simulink model "exSyncGenPVinv_sim"  (R2014b)
settings: Solver=ode45  SolverMode=SingleTasking  StartTime=0.0  StopTime=20  MaxStep=0.002  RelTol=1e-07
values from neighbouring files (symbols this model uses):
  bus1_vd = 2^0.5*1e3    (= 1414.21356237)    [ex3busPV.m]    (also in exLongLinePV.m = 141421.356237)
  Cbus_ext = 1e6*mpcC.bus(ssgen,BS)./(ws*baseV(ssgen).^2)    [exDroopA.m]    (also in exDroopB.m; exSyncGenPVinv.m)
  Cbuseff = 2*Ebus/Vdcset^2    [exSyncGenPVinv.m]
  droop_D = 5e-4*(2/poles)./J    [exSyncGenPVinv.m]
  droop_Pref = 0.25*Pbase    (= 75000000)    [ex7busLongLine.m]    (also in exDroopA.m = mpc.gen(2:end,PG)*1e6; exDroopB.m = mpc.gen(:,PG)*1e6; exSyncGenPVinv.m = droop_Pref( [1:(synrp-1),(synrp+1):end]  ))
  If_dc = 0.2*Prt./Ert    [ex14busSGandPV.m]    (also in ex7busLongLine.m = Prt./(60*Vf_dc); exDroopA.m = Prt./(60*Vf_dc); exDroopB.m = Prt./(60*Vf_dc); exSyncGenPVinv.m)
  Kci = Kcp^2/(2*Linv)    [exSyncGenPVinv.m]    (also in pv_dq.m = 3.11562907794)
  Kcp = 10*4*pi*Linv    [exSyncGenPVinv.m]    (also in pv_dq.m = 0.0495867768595)
  Kpi = 0.1*Kpp^2/(Ebus/Vinv_rt)    [exSyncGenPVinv.m]    (also in pv_dq.m = 251.934662919)
  Kpp = 200*(Ebus/Vinv_rt)    [exSyncGenPVinv.m]    (also in pv_dq.m = 12.596733146)
  L0 = 0.1*Ld    [ex14busSGandPV.m]    (also in ex7busLongLine.m; exDroopA.m; exDroopB.m; exSyncGenPVinv.m)
  Laf = (2^0.5)*Ert./(ws*If_dc)    [ex14busSGandPV.m]    (also in ex7busLongLine.m; exDroopA.m; exDroopB.m; exSyncGenPVinv.m = (2^0.5)*5*Ert.^2./(ws*Prt))
  Lb2 = 2*Ld.*Lff - 3*Laf.^2    [ex14busSGandPV.m]    (also in ex7busLongLine.m; exDroopA.m; exDroopB.m; exSyncGenPVinv.m)
  Ld = 0.6*Lpu    [ex14busSGandPV.m]    (also in ex7busLongLine.m = 0.3*Lpu; exDroopA.m = 0.3*Lpu; exDroopB.m = 0.3*Lpu; exSyncGenPVinv.m)
  Lff = 2*Laf.^2./Ld    [ex14busSGandPV.m]    (also in ex7busLongLine.m; exDroopA.m; exDroopB.m; exSyncGenPVinv.m)
  Linv = 10*(1/ws)*Pinv_rt/Vinv_rt^2    [exSyncGenPVinv.m]
  Lq = Ld    [ex14busSGandPV.m]    (also in ex7busLongLine.m; exDroopA.m; exDroopB.m; exSyncGenPVinv.m)
  nG = length(ssgen)    [exDroopA.m]    (also in exSyncGenPVinv.m)
  Pdc_op = 0.6*Pinv_rt    [exSyncGenPVinv.m]    (also in pv_dq.m = 1600000)
  poles_2Jws = poles./(2*J*ws)    [ex14busSGandPV.m]    (also in ex2busStability.m = poles./(2*ws*J); ex7busLongLine.m; ex9busSG.m = poles./(2*ws*J); exDroopA.m)
  Qstar = 0    [exSyncGenPVinv.m]    (also in pv_dq.m)
  Ra = 0.05*Ert.^2./Prt    [ex14busSGandPV.m]    (also in ex7busLongLine.m = 0.01*Ert.^2./Prt; exDroopA.m = 0.01*Ert.^2./Prt; exDroopB.m = 0.01*Ert.^2./Prt; exSyncGenPVinv.m)
  Rf = Lff/1.2    [ex14busSGandPV.m]    (also in ex7busLongLine.m = Vf_dc./If_dc; exDroopA.m = Vf_dc./If_dc; exDroopB.m = Vf_dc./If_dc; exSyncGenPVinv.m)
  synrp = 2    [exSyncGenPVinv.m]
  units_to_net = zeros(1,3*Nss)    [ex14busSGandPV.m]    (also in exDroopA.m = [1,4:(3+nG),2,(4+nG):(3+2*nG),3,(4+2*nG):(3+3*nG)]; exSyncGenPVinv.m = [1,4:(3+nG),2,(4+nG):(3+2*nG),3,(4+2*nG):(3+3*nG)])
  vcap_init_0 = 0*vppa    [exDroopA.m]    (also in exDroopB.m; exSyncGenPVinv.m)
  vcap_init_d = real(vppa)    [exDroopA.m]    (also in exDroopB.m; exSyncGenPVinv.m)
  vcap_init_q = imag(vppa)    [exDroopA.m]    (also in exDroopB.m; exSyncGenPVinv.m)
  Vdcset = (2^0.5)*Vinv_rt/duty_max    [exSyncGenPVinv.m]    (also in pv_dq.m = 19958.8053116)
  Vf_dc = If_dc.*Rf    [ex14busSGandPV.m]    (also in ex7busLongLine.m = 500 * ones(size(Ert)); exDroopA.m = 500 * ones(size(Ert)); exDroopB.m = 500 * ones(size(Ert)); exSyncGenPVinv.m)
  vinf_0 = 0    [ex14busSGandPV.m]    (also in ex7busLongLine.m; exDroopA.m; exSyncGenPVinv.m)
  vinf_d = (2^0.5)*mpcA.bus(1,VM)*baseV    [ex14busSGandPV.m]    (also in ex7busLongLine.m = 250457.221896; exDroopA.m = (2^0.5)*mpc.bus(1,VM)*baseV(1); exSyncGenPVinv.m = (2^0.5)*mpc.bus(1,VM)*baseV(1))
  vinf_q = 0    [ex14busSGandPV.m]    (also in ex7busLongLine.m; exDroopA.m; exSyncGenPVinv.m)
  Vinv_rt = mpc.bus(ssgen(synrp),VM).*baseV(ssgen(synrp))    [exSyncGenPVinv.m]    (also in pv_dq.m = 12701.7059222)
  ws = 2*pi*50    (= 314.159265359)    [ex14busSGandPV.m]    (also in ex2busStability.m; ex3busPV.m; ex7busLongLine.m; ex9busSG.m)
undefined symbols (not defined in the file or in its folder): Anet, Bnet, Cnet, Dnet, full, magnitude, net_to_units
libraries: simulink x1
settings Model: Creator=COPEC  LastModifiedBy=yoashl
settings OptimizationCC: BlockReduction=off  BooleanDataType=off
settings DebuggingCC: SaveWithParameterizedLinksMsg=none  UnderspecifiedInitializationDetection=Classic  MergeDetectMultiDrivingBlocksExec=none  SignalResolutionControl=TryResolveAllWithWarning  SolverPrmCheckMsg=none  FrameProcessingCompatibilityMsg=error
settings HardwareCC: TargetUnknown=on

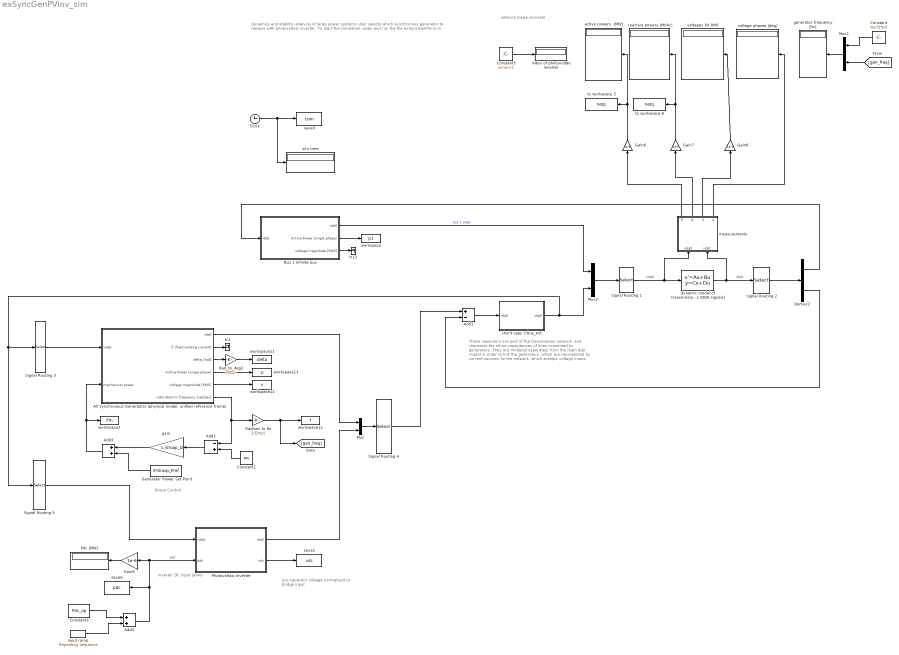
== system exSyncGenPVinv_sim ==
  note: Droop Control
  note: Dynamics and stability analysis of large power systems
      | User selects which synchronous generator to replace with photovoltaic inverter.
      |
      | To start the simulation, open and run the file
      | exSyncGenPVinv.m
  note: These capacitors are part of the transmission network, and represent the shunt capacitances of lines connected to generators. They are modeled seperately from the main dq0 model in order to link the generators, which are represented by current sources, to the network, which accepts voltage inputs.
  note: network measurements
  note: bus capacitor voltage normalized to bridge input
  note: inverter DC input power
  Add1 : Sum  Inputs=+-
  Add2 : Sum  Inputs=-+
  Add3 : Sum
  Add4 : Sum
  "All Synchronous Generators (physical model, unified reference frame)" : Subsystem
  Bus 1 Infinite bus : Subsystem
  Clock : Clock
  Constant : Constant  Value=ws/(2*pi)
  Constant1 : Constant  Value=ws
  Constant2 : Constant  Value=Pdc_op
  Constant3 : Constant  Value=synrp+1
  Demux2 : Demux  Outputs=[3 , length(net_to_units)-3]
  Gain6 : Gain  Gain=1e-6
  Gain7 : Gain  Gain=1e-6
  Gain8 : Gain  Gain=1e-3
  Gain9 : Gain  Gain=1e-6
  Generator Power Set Point : Constant  Value=3*droop_Pref
  Mux : Mux  Inputs=2
  Mux1 : Mux  Inputs=2
  Mux2 : Mux  Inputs=2
  Pdc [MW] : Display
  Photovoltaic Inverter : Subsystem
  Rad/sec to Hz : Gain  Gain=1/(2*pi)
  Rad_to_deg2 : Gain  Gain=180/pi
  Signal Routing 1 : Selector  InputPortWidth=length(units_to_net)  IndexOptions=Index vector (dialog)  Indices=units_to_net  OutputSizes=1
  Signal Routing 2 : Selector  InputPortWidth=length(net_to_units)  IndexOptions=Index vector (dialog)  Indices=net_to_units  OutputSizes=1
  Signal Routing 3 : Selector  InputPortWidth=3*nG  IndexOptions=Index vector (dialog)  Indices=routing1  OutputSizes=1
  Signal Routing 4 : Selector  InputPortWidth=3*nG  IndexOptions=Index vector (dialog)  Indices=routing3  OutputSizes=1
  Signal Routing 5 : Selector  InputPortWidth=3*nG  IndexOptions=Index vector (dialog)  Indices=routing2  OutputSizes=1
  active powers  [MW] : Display
  dynamic model of transmission network with integrated loads (DQ0 signals) : StateSpace  A=full(Anet)  B=full(Bnet)  C=full(Cnet)  D=full(Dnet)  X0=0
  gain : Gain  Gain=1./droop_D
  generator frequency [Hz] : Display
  index of photovoltaic inverter : Display
  input ramp : simulink/Sources/Repeating Sequence  rep_seq_t=[0 1 1e6]  rep_seq_y=[0 0 0]
  measurements : Subsystem
  reactive powers [MVAr] : Display
  save0 : ToWorkspace  VariableName=tsim  SampleTime=-1
  save2 : ToWorkspace  VariableName=vdc  SampleTime=-1
  save6 : ToWorkspace  VariableName=pdc  SampleTime=-1
  "shunt caps 'Cbus_ext' " : Subsystem
  sim time : Display
  to workspace 5 : ToWorkspace  VariableName=netp  SampleTime=-1
  to workspace 6 : ToWorkspace  VariableName=netq  SampleTime=-1
  tr12 : Terminator
  tr2 : Terminator
  voltage phases [deg] : Display
  voltages kV RMS : Display
  workspace : ToWorkspace  VariableName=p1  SampleTime=-1
  workspace1 : ToWorkspace  VariableName=Pm  SampleTime=-1
  workspace11 : ToWorkspace  VariableName=delta  SampleTime=-1
  workspace12 : ToWorkspace  VariableName=f  SampleTime=-1
  workspace13 : ToWorkspace  VariableName=p  SampleTime=-1
  workspace14 : ToWorkspace  VariableName=v  SampleTime=-1
  wires:
  Clock/1 -> sim time/1, save0/1
  Bus 1 Infinite bus/3(voltage magnitude [RMS]) -> tr12/1
  Bus 1 Infinite bus/2(Active Power (single phase)) -> workspace/1
  "All Synchronous Generators (physical model, unified reference frame)"/2(if (field winding current)) -> tr2/1
  "All Synchronous Generators (physical model, unified reference frame)"/3(delta_[rad]) -> Rad_to_deg2/1
  Rad_to_deg2/1 -> workspace11/1
  "All Synchronous Generators (physical model, unified reference frame)"/6(rotor electric frequency [rad/sec]) -> Rad/sec to Hz/1, Add2/1
  Rad/sec to Hz/1 -> workspace12/1, [gen_freq]
  "All Synchronous Generators (physical model, unified reference frame)"/4(Active Power (single phase)) -> workspace13/1
  "All Synchronous Generators (physical model, unified reference frame)"/5(voltage magnitude [RMS]) -> workspace14/1
  Add1/1 -> "shunt caps 'Cbus_ext' "/1(idq0)
  "shunt caps 'Cbus_ext' "/1(vdq0) -> Signal Routing 5/1, Signal Routing 3/1, Mux2/2
  Bus 1 Infinite bus/1(vdq0) -> Mux2/1  "bus 1 vdq0"
  Mux2/1 -> Signal Routing 1/1
  Signal Routing 1/1 -> measurements/1(vdq0), dynamic model of transmission network with integrated loads (DQ0 signals)/1  "vdq0"
  dynamic model of transmission network with integrated loads (DQ0 signals)/1 -> measurements/2(idq0), Signal Routing 2/1  "idq0"
  Signal Routing 2/1 -> Demux2/1
  Demux2/2 -> Add1/2
  Demux2/1 -> Bus 1 Infinite bus/1(idq0)
  Constant1/1 -> Add2/2
  Add2/1 -> gain/1
  Generator Power Set Point/1 -> Add3/2
  gain/1 -> Add3/1
  Add3/1 -> workspace1/1, "All Synchronous Generators (physical model, unified reference frame)"/2(mechanical power)
  Gain8/1 -> voltages kV RMS/1
  measurements/2(Q) -> Gain7/1
  Constant/1 -> Mux1/1
  Gain7/1 -> reactive powers [MVAr]/1, to workspace 6/1
  Mux1/1 -> generator frequency [Hz]/1
  measurements/3(Vm_RMS) -> Gain8/1
  measurements/4(Vph_deg) -> voltage phases [deg]/1
  Gain6/1 -> to workspace 5/1, active powers  [MW]/1
  [gen_freq] -> Mux1/2
  measurements/1(P) -> Gain6/1
  Photovoltaic Inverter/2(vdc) -> save2/1
  input ramp/1 -> Add4/2
  Add4/1 -> Photovoltaic Inverter/2(pdc), Gain9/1, save6/1  "pdc"
  Gain9/1 -> Pdc [MW]/1
  Constant2/1 -> Add4/1
  "All Synchronous Generators (physical model, unified reference frame)"/1(idq0) -> Mux/1
  Signal Routing 3/1 -> "All Synchronous Generators (physical model, unified reference frame)"/1(vdq0)
  Photovoltaic Inverter/1(idq0) -> Mux/2
  Mux/1 -> Signal Routing 4/1
  Signal Routing 4/1 -> Add1/1
  Signal Routing 5/1 -> Photovoltaic Inverter/1(vdq0)
  Constant3/1 -> index of photovoltaic inverter/1

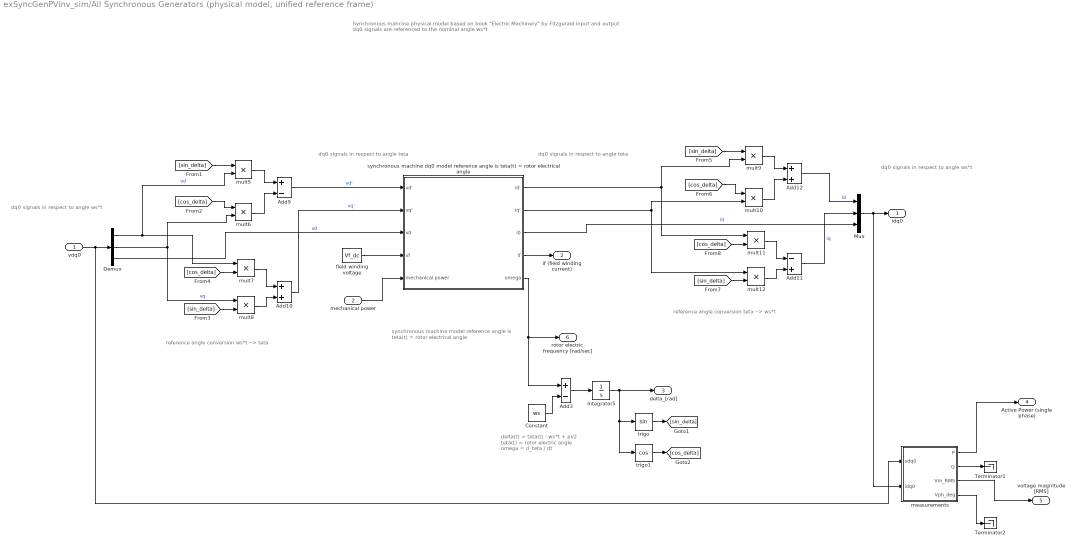
== system exSyncGenPVinv_sim/All Synchronous Generators (physical model, unified reference frame) ==
  note: Synchronous mahcine physical model
      | based on book "Electric Machinery" by Fitzgerald
      |
      | input and output dq0 signals are referenced
      | to the nominal angle ws*t
  note: reference angle conversion ws*t --> teta
  note: synchronous machine model
      | reference angle is
      | teta(t) = rotor electrical angle
  note: reference angle conversion teta --> ws*t
  note: dq0 signals in respect to angle ws*t
  note: dq0 signals in respect to angle ws*t
  note: dq0 signals in respect to angle teta
  note: dq0 signals in respect to angle teta
  note: delta(t) = teta(t) - ws*t + pi/2
      | teta(t) = rotor electric angle
      | omega = d_teta / dt
  vdq0 : Inport
  mechanical power : Inport  Port=2
  Add10 : Sum
  Add11 : Sum  Inputs=-+
  Add12 : Sum
  Add3 : Sum  Inputs=+-
  Add9 : Sum  Inputs=+-
  Constant : Constant  Value=ws
  Demux : Demux  Outputs=3
  Integrator5 : Integrator
  Mux : Mux  Inputs=3
  Terminator1 : Terminator
  Terminator2 : Terminator
  field winding voltage : Constant  Value=Vf_dc
  measurements : Subsystem
  mult{5..12} (8 alike) : Product  Inputs=**
  synchronous machine dq0 model reference angle is teta(t) = rotor electrical angle : Subsystem
  trigo : Trigonometry
  trigo1 : Trigonometry  Operator=cos
  idq0 : Outport
  if (field winding current) : Outport  Port=2
  delta_[rad] : Outport  Port=3
  Active Power (single phase) : Outport  Port=4
  voltage magnitude [RMS] : Outport  Port=5
  rotor electric frequency [rad/sec] : Outport  Port=6
  wires:
  vdq0/1 -> measurements/1(vdq0), Demux/1
  Demux/1 -> mult5/2, mult7/1  "vd"
  Demux/2 -> mult6/2, mult8/1  "vq"
  mult5/1 -> Add9/1
  mult6/1 -> Add9/2
  [sin_delta] -> mult5/1
  [cos_delta] -> mult6/1
  mult7/1 -> Add10/1
  mult8/1 -> Add10/2
  [cos_delta] -> mult7/2
  [sin_delta] -> mult8/2
  mult9/1 -> Add12/1
  mult10/1 -> Add12/2
  [sin_delta] -> mult9/1
  [cos_delta] -> mult10/1
  mult11/1 -> Add11/1
  mult12/1 -> Add11/2
  [cos_delta] -> mult11/2
  [sin_delta] -> mult12/2
  Mux/1 -> measurements/2(idq0), idq0/1
  Add11/1 -> Mux/2  "iq"
  Add12/1 -> Mux/1  "id"
  synchronous machine dq0 model reference angle is teta(t) = rotor electrical angle/1(id') -> mult11/1, mult9/2
  synchronous machine dq0 model reference angle is teta(t) = rotor electrical angle/2(iq') -> mult12/1, mult10/2
  Add9/1 -> synchronous machine dq0 model reference angle is teta(t) = rotor electrical angle/1(vd')  "vd'"
  mechanical power/1 -> synchronous machine dq0 model reference angle is teta(t) = rotor electrical angle/5(mechanical power)
  Demux/3 -> synchronous machine dq0 model reference angle is teta(t) = rotor electrical angle/3(v0)  "v0"
  Add10/1 -> synchronous machine dq0 model reference angle is teta(t) = rotor electrical angle/2(vq')  "vq'"
  field winding voltage/1 -> synchronous machine dq0 model reference angle is teta(t) = rotor electrical angle/4(vf)
  synchronous machine dq0 model reference angle is teta(t) = rotor electrical angle/3(i0) -> Mux/3  "i0"
  synchronous machine dq0 model reference angle is teta(t) = rotor electrical angle/4(if) -> if (field winding current)/1
  trigo/1 -> [sin_delta]
  trigo1/1 -> [cos_delta]
  Add3/1 -> Integrator5/1
  Constant/1 -> Add3/2
  synchronous machine dq0 model reference angle is teta(t) = rotor electrical angle/5(omega) -> Add3/1, rotor electric frequency [rad/sec]/1
  Integrator5/1 -> delta_[rad]/1, trigo1/1, trigo/1
  measurements/1(P) -> Active Power (single phase)/1
  measurements/2(Q) -> Terminator1/1
  measurements/3(Vm_RMS) -> voltage magnitude [RMS]/1
  measurements/4(Vph_deg) -> Terminator2/1

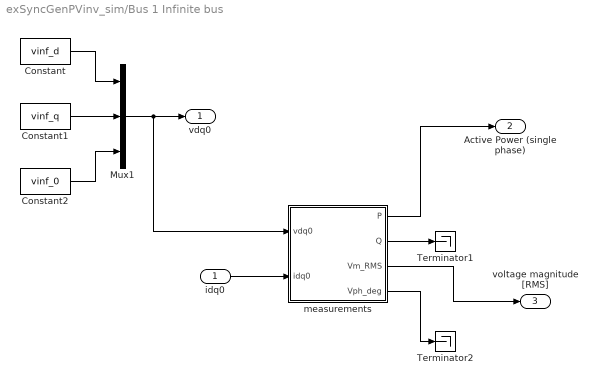
== system exSyncGenPVinv_sim/Bus 1 Infinite bus ==
  idq0 : Inport
  Constant : Constant  Value=vinf_d
  Constant1 : Constant  Value=vinf_q
  Constant2 : Constant  Value=vinf_0
  Mux1 : Mux  Inputs=3
  Terminator1 : Terminator
  Terminator2 : Terminator
  measurements : Subsystem
  vdq0 : Outport
  Active Power (single phase) : Outport  Port=2
  voltage magnitude [RMS] : Outport  Port=3
  wires:
  measurements/1(P) -> Active Power (single phase)/1
  measurements/2(Q) -> Terminator1/1
  measurements/3(Vm_RMS) -> voltage magnitude [RMS]/1
  measurements/4(Vph_deg) -> Terminator2/1
  idq0/1 -> measurements/2(idq0)
  Mux1/1 -> measurements/1(vdq0), vdq0/1
  Constant/1 -> Mux1/1
  Constant1/1 -> Mux1/2
  Constant2/1 -> Mux1/3

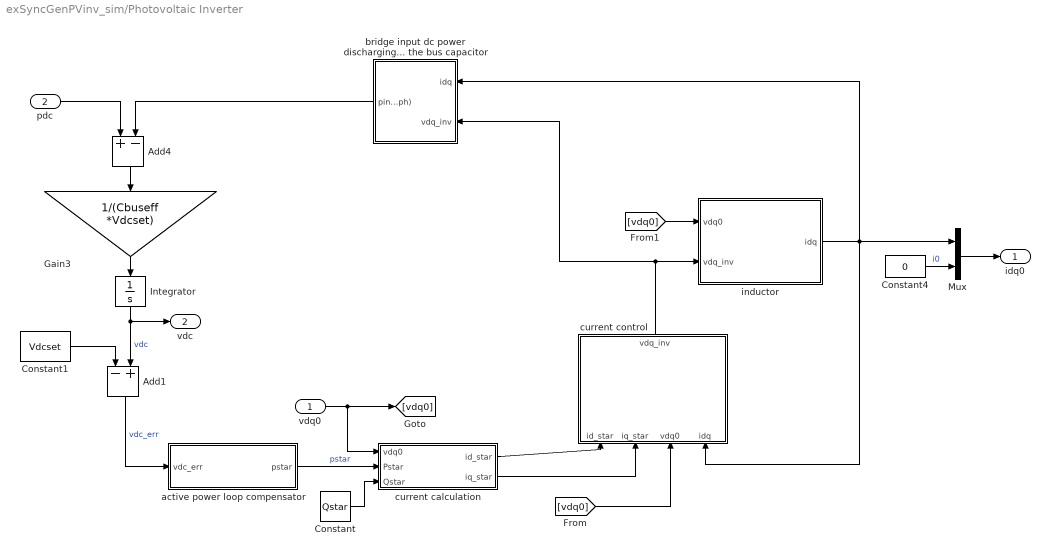
== system exSyncGenPVinv_sim/Photovoltaic Inverter ==
  vdq0 : Inport
  pdc : Inport  Port=2
  Add1 : Sum  Inputs=-+
  Add4 : Sum  Inputs=+-
  Constant : Constant  Value=Qstar
  Constant1 : Constant  Value=Vdcset
  Constant4 : Constant  Value=0
  Gain3 : Gain  Gain=1/(Cbuseff *Vdcset)
  Integrator : Integrator  InitialCondition=Vdcset
  Mux : Mux  Inputs=2
  active power loop compensator : Subsystem
  bridge input dc power discharging the bus capacitor : Subsystem
  current control : Subsystem
  current calculation : Subsystem
  inductor : Subsystem
  idq0 : Outport
  vdc : Outport  Port=2
  wires:
  Integrator/1 -> Add1/2, vdc/1  "vdc"
  Constant/1 -> current calculation/3(Qstar)
  Add4/1 -> Gain3/1
  Constant1/1 -> Add1/1
  active power loop compensator/1(pstar) -> current calculation/2(Pstar)  "pstar"
  Gain3/1 -> Integrator/1
  current calculation/2(iq_star) -> current control/2(iq_star)
  current calculation/1(id_star) -> current control/1(id_star)
  Add1/1 -> active power loop compensator/1(vdc_err)  "vdc_err"
  pdc/1 -> Add4/1
  vdq0/1 -> current calculation/1(vdq0), [vdq0]
  [vdq0] -> current control/3(vdq0)
  [vdq0] -> inductor/1(vdq0)
  current control/1(vdq_inv) -> bridge input dc power discharging the bus capacitor/2(vdq_inv), inductor/2(vdq_inv)
  bridge input dc power discharging the bus capacitor/1(pinv (3ph)) -> Add4/2
  Mux/1 -> idq0/1
  inductor/1(idq) -> bridge input dc power discharging the bus capacitor/1(idq), Mux/1, current control/4(idq)
  Constant4/1 -> Mux/2  "i0"

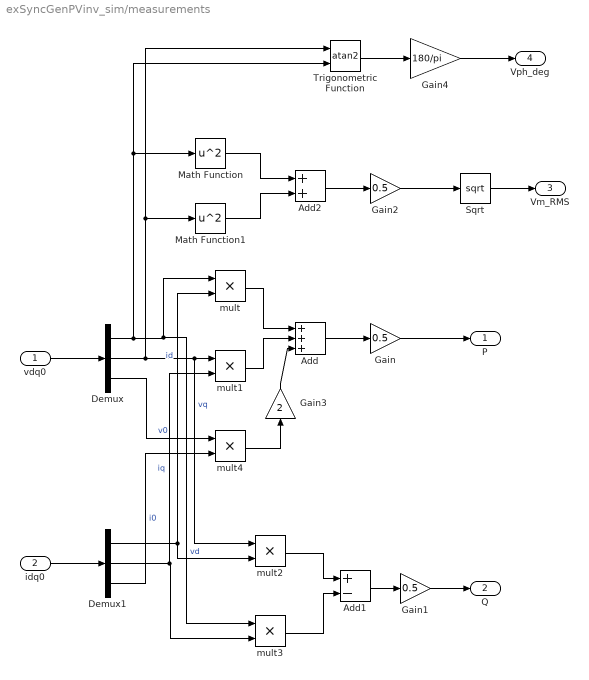
== system exSyncGenPVinv_sim/measurements ==
  vdq0 : Inport
  idq0 : Inport  Port=2
  Add : Sum  Inputs=+++
  Add1 : Sum  Inputs=+-
  Add2 : Sum
  Demux : Demux  Outputs=3
  Demux1 : Demux  Outputs=3
  Gain : Gain  Gain=0.5
  Gain1 : Gain  Gain=0.5
  Gain2 : Gain  Gain=0.5
  Gain3 : Gain  Gain=2
  Gain4 : Gain  Gain=180/pi
  Math Function : Math  Operator=square  SaturateOnIntegerOverflow=on
  Math Function1 : Math  Operator=square  SaturateOnIntegerOverflow=on
  Sqrt : Sqrt  SaturateOnIntegerOverflow=on
  Trigonometric Function : Trigonometry  Operator=atan2
  mult{,1..4} (5 alike) : Product  Inputs=**
  P : Outport
  Q : Outport  Port=2
  Vm_RMS : Outport  Port=3
  Vph_deg : Outport  Port=4
  wires:
  idq0/1 -> Demux1/1
  vdq0/1 -> Demux/1
  Demux/1 -> Math Function/1, Trigonometric Function/2, mult3/1, mult/1  "vd"
  Demux/2 -> Trigonometric Function/1, Math Function1/1, mult2/1, mult1/1  "vq"
  Demux1/1 -> mult/2, mult2/2  "id"
  Demux1/2 -> mult3/2, mult1/2  "iq"
  Demux/3 -> mult4/1  "v0"
  Demux1/3 -> mult4/2  "i0"
  mult/1 -> Add/1
  mult1/1 -> Add/2
  Add/1 -> Gain/1
  mult2/1 -> Add1/1
  mult3/1 -> Add1/2
  Add1/1 -> Gain1/1
  Sqrt/1 -> Vm_RMS/1
  Math Function/1 -> Add2/1
  Math Function1/1 -> Add2/2
  Add2/1 -> Gain2/1
  Gain2/1 -> Sqrt/1
  Gain/1 -> P/1
  Gain1/1 -> Q/1
  mult4/1 -> Gain3/1
  Gain3/1 -> Add/3
  Trigonometric Function/1 -> Gain4/1
  Gain4/1 -> Vph_deg/1

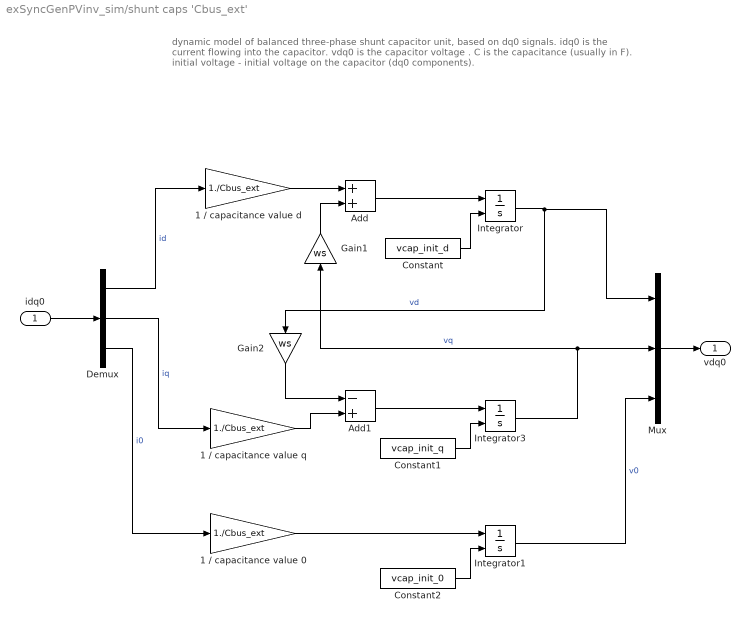
== system exSyncGenPVinv_sim/shunt caps 'Cbus_ext'  ==
  note: dynamic model of balanced three-phase shunt capacitor unit, based on dq0 signals.
      | idq0 is the current flowing into the capacitor.
      | vdq0 is the capacitor voltage .
      | C is the capacitance (usually in F).
      | initial voltage - initial voltage on the capacitor (dq0 components).
  idq0 : Inport
  1 / capacitance value 0 : Gain  Gain=1./Cbus_ext
  1 / capacitance value d : Gain  Gain=1./Cbus_ext
  1 / capacitance value q : Gain  Gain=1./Cbus_ext
  Add : Sum
  Add1 : Sum  Inputs=-+
  Constant : Constant  Value=vcap_init_d
  Constant1 : Constant  Value=vcap_init_q
  Constant2 : Constant  Value=vcap_init_0
  Demux : Demux  Outputs=3
  Gain1 : Gain  Gain=ws
  Gain2 : Gain  Gain=ws
  Integrator : Integrator  InitialConditionSource=external  InitialCondition=bus1_vd
  Integrator1 : Integrator  InitialConditionSource=external  InitialCondition=bus1_vd
  Integrator3 : Integrator  InitialConditionSource=external  InitialCondition=bus1_vd
  Mux : Mux  Inputs=3
  vdq0 : Outport
  wires:
  Integrator1/1 -> Mux/3  "v0"
  Mux/1 -> vdq0/1
  Integrator/1 -> Gain2/1, Mux/1  "vd"
  Integrator3/1 -> Gain1/1, Mux/2  "vq"
  Add/1 -> Integrator/1
  Gain1/1 -> Add/2
  idq0/1 -> Demux/1
  1 / capacitance value d/1 -> Add/1
  Add1/1 -> Integrator3/1
  Gain2/1 -> Add1/1
  1 / capacitance value q/1 -> Add1/2
  1 / capacitance value 0/1 -> Integrator1/1
  Constant/1 -> Integrator/2
  Constant1/1 -> Integrator3/2
  Constant2/1 -> Integrator1/2
  Demux/1 -> 1 / capacitance value d/1  "id"
  Demux/2 -> 1 / capacitance value q/1  "iq"
  Demux/3 -> 1 / capacitance value 0/1  "i0"

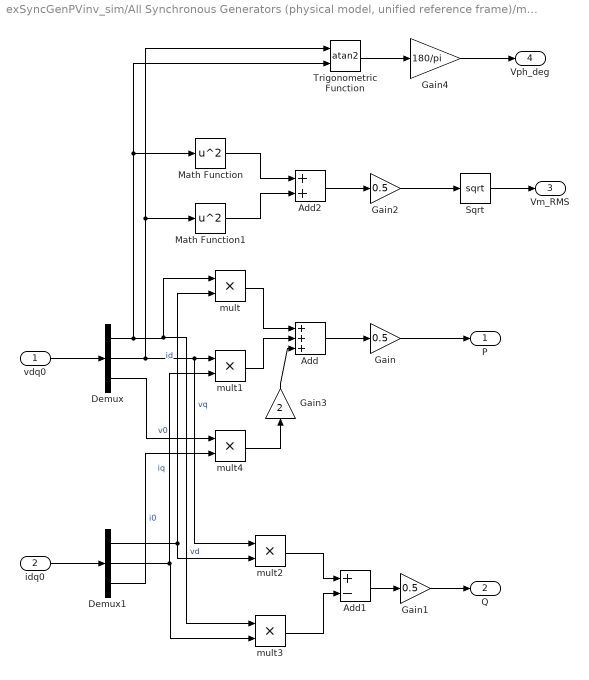
== system exSyncGenPVinv_sim/All Synchronous Generators (physical model, unified reference frame)/measurements ==
  vdq0 : Inport
  idq0 : Inport  Port=2
  Add : Sum  Inputs=+++
  Add1 : Sum  Inputs=+-
  Add2 : Sum
  Demux : Demux  Outputs=3
  Demux1 : Demux  Outputs=3
  Gain : Gain  Gain=0.5
  Gain1 : Gain  Gain=0.5
  Gain2 : Gain  Gain=0.5
  Gain3 : Gain  Gain=2
  Gain4 : Gain  Gain=180/pi
  Math Function : Math  Operator=square  SaturateOnIntegerOverflow=on
  Math Function1 : Math  Operator=square  SaturateOnIntegerOverflow=on
  Sqrt : Sqrt  SaturateOnIntegerOverflow=on
  Trigonometric Function : Trigonometry  Operator=atan2
  mult{,1..4} (5 alike) : Product  Inputs=**
  P : Outport
  Q : Outport  Port=2
  Vm_RMS : Outport  Port=3
  Vph_deg : Outport  Port=4
  wires:
  idq0/1 -> Demux1/1
  vdq0/1 -> Demux/1
  Demux/1 -> Math Function/1, Trigonometric Function/2, mult3/1, mult/1  "vd"
  Demux/2 -> Trigonometric Function/1, Math Function1/1, mult2/1, mult1/1  "vq"
  Demux1/1 -> mult/2, mult2/2  "id"
  Demux1/2 -> mult3/2, mult1/2  "iq"
  Demux/3 -> mult4/1  "v0"
  Demux1/3 -> mult4/2  "i0"
  mult/1 -> Add/1
  mult1/1 -> Add/2
  Add/1 -> Gain/1
  mult2/1 -> Add1/1
  mult3/1 -> Add1/2
  Add1/1 -> Gain1/1
  Sqrt/1 -> Vm_RMS/1
  Math Function/1 -> Add2/1
  Math Function1/1 -> Add2/2
  Add2/1 -> Gain2/1
  Gain2/1 -> Sqrt/1
  Gain/1 -> P/1
  Gain1/1 -> Q/1
  mult4/1 -> Gain3/1
  Gain3/1 -> Add/3
  Trigonometric Function/1 -> Gain4/1
  Gain4/1 -> Vph_deg/1

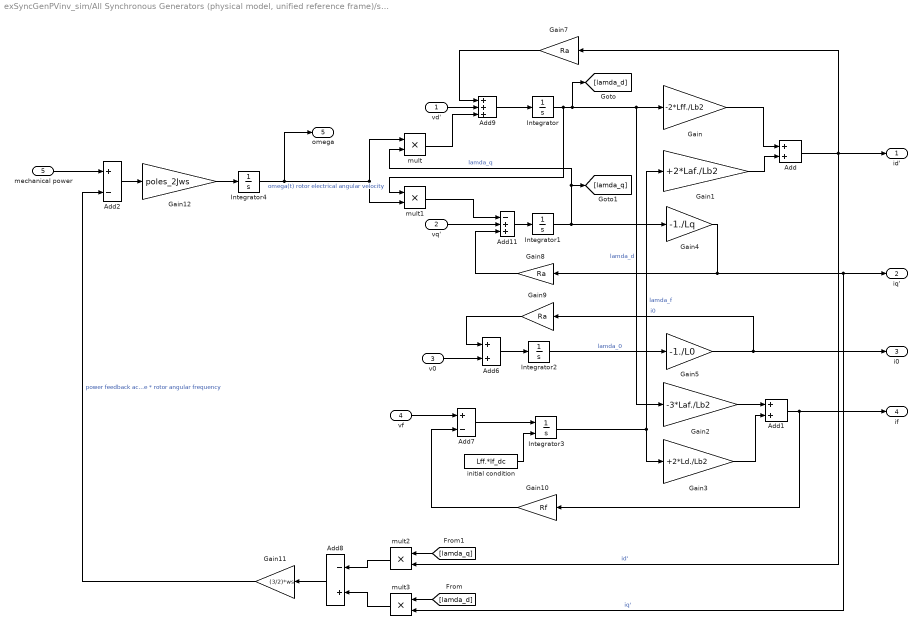
== system exSyncGenPVinv_sim/All Synchronous Generators (physical model, unified reference frame)/synchronous machine dq0 model reference angle is teta(t) = rotor electrical angle ==
  vd' : Inport
  vq' : Inport  Port=2
  v0 : Inport  Port=3
  vf : Inport  Port=4
  mechanical power : Inport  Port=5
  Add : Sum
  Add1 : Sum
  Add11 : Sum  Inputs=-++
  Add2 : Sum  Inputs=+-
  Add6 : Sum
  Add7 : Sum  Inputs=+-
  Add8 : Sum  Inputs=-+
  Add9 : Sum  Inputs=+++
  Gain : Gain  Gain=-2*Lff./Lb2
  Gain1 : Gain  Gain=+2*Laf./Lb2
  Gain10 : Gain  Gain=Rf
  Gain11 : Gain  Gain=(3/2)*ws
  Gain12 : Gain  Gain=poles_2Jws
  Gain2 : Gain  Gain=-3*Laf./Lb2
  Gain3 : Gain  Gain=+2*Ld./Lb2
  Gain4 : Gain  Gain=-1./Lq
  Gain5 : Gain  Gain=-1./L0
  Gain7 : Gain  Gain=Ra
  Gain8 : Gain  Gain=Ra
  Gain9 : Gain  Gain=Ra
  Integrator : Integrator
  Integrator1 : Integrator
  Integrator2 : Integrator
  Integrator3 : Integrator  InitialConditionSource=external  InitialCondition=Lff(1)*If_dc(1)
  Integrator4 : Integrator  InitialCondition=ws
  initial condition : Constant  Value=Lff.*If_dc
  mult{,1..3} (4 alike) : Product  Inputs=**
  id' : Outport
  iq' : Outport  Port=2
  i0 : Outport  Port=3
  if : Outport  Port=4
  omega : Outport  Port=5
  wires:
  Gain1/1 -> Add/2
  Add6/1 -> Integrator2/1
  mechanical power/1 -> Add2/1
  Integrator/1 -> mult1/1, Gain2/1, Gain/1, [lamda_d]  "lamda_d"
  Gain5/1 -> i0/1, Gain9/1  "i0"
  Integrator1/1 -> Gain4/1, [lamda_q], mult/2  "lamda_q"
  Integrator2/1 -> Gain5/1  "lamda_0"
  Integrator3/1 -> Gain1/1, Gain3/1  "lamda_f"
  Add1/1 -> if/1, Gain10/1
  Gain4/1 -> iq'/1, mult3/2, Gain8/1  "iq'"
  Add/1 -> mult2/2, id'/1, Gain7/1  "id'"
  Gain/1 -> Add/1
  vf/1 -> Add7/1
  Add7/1 -> Integrator3/1
  Gain9/1 -> Add6/1
  Add8/1 -> Gain11/1
  Gain11/1 -> Add2/2  "power feedback acting to slow the rotor = Torque * rotor angular frequency"
  Gain8/1 -> Add11/3
  mult/1 -> Add9/3
  mult1/1 -> Add11/1
  Add9/1 -> Integrator/1
  vd'/1 -> Add9/2
  Gain3/1 -> Add1/2
  Gain2/1 -> Add1/1
  Gain10/1 -> Add7/2
  Add11/1 -> Integrator1/1
  Gain7/1 -> Add9/1
  mult3/1 -> Add8/2
  mult2/1 -> Add8/1
  v0/1 -> Add6/2
  vq'/1 -> Add11/2
  [lamda_q] -> mult2/1
  [lamda_d] -> mult3/1
  Integrator4/1 -> omega/1, mult1/2, mult/1  "omega(t) rotor electrical angular velocity"
  Add2/1 -> Gain12/1
  Gain12/1 -> Integrator4/1
  initial condition/1 -> Integrator3/2

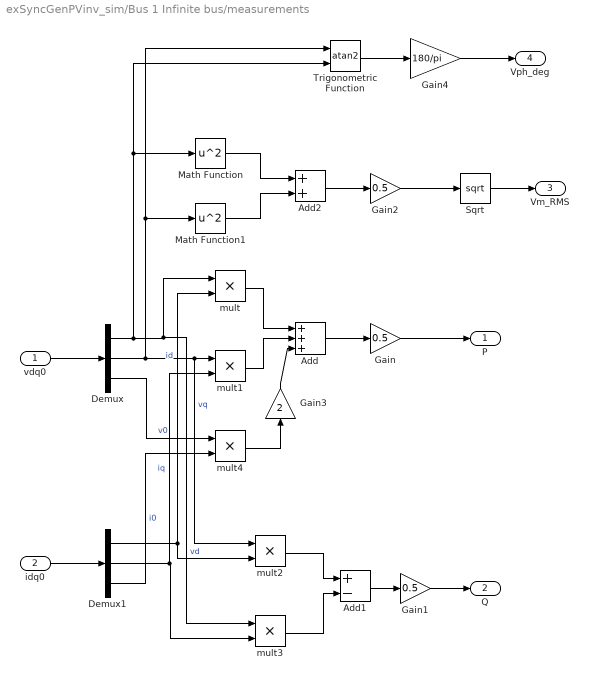
== system exSyncGenPVinv_sim/Bus 1 Infinite bus/measurements ==
  vdq0 : Inport
  idq0 : Inport  Port=2
  Add : Sum  Inputs=+++
  Add1 : Sum  Inputs=+-
  Add2 : Sum
  Demux : Demux  Outputs=3
  Demux1 : Demux  Outputs=3
  Gain : Gain  Gain=0.5
  Gain1 : Gain  Gain=0.5
  Gain2 : Gain  Gain=0.5
  Gain3 : Gain  Gain=2
  Gain4 : Gain  Gain=180/pi
  Math Function : Math  Operator=square  SaturateOnIntegerOverflow=on
  Math Function1 : Math  Operator=square  SaturateOnIntegerOverflow=on
  Sqrt : Sqrt  SaturateOnIntegerOverflow=on
  Trigonometric Function : Trigonometry  Operator=atan2
  mult{,1..4} (5 alike) : Product  Inputs=**
  P : Outport
  Q : Outport  Port=2
  Vm_RMS : Outport  Port=3
  Vph_deg : Outport  Port=4
  wires:
  idq0/1 -> Demux1/1
  vdq0/1 -> Demux/1
  Demux/1 -> Math Function/1, Trigonometric Function/2, mult3/1, mult/1  "vd"
  Demux/2 -> Trigonometric Function/1, Math Function1/1, mult2/1, mult1/1  "vq"
  Demux1/1 -> mult/2, mult2/2  "id"
  Demux1/2 -> mult3/2, mult1/2  "iq"
  Demux/3 -> mult4/1  "v0"
  Demux1/3 -> mult4/2  "i0"
  mult/1 -> Add/1
  mult1/1 -> Add/2
  Add/1 -> Gain/1
  mult2/1 -> Add1/1
  mult3/1 -> Add1/2
  Add1/1 -> Gain1/1
  Sqrt/1 -> Vm_RMS/1
  Math Function/1 -> Add2/1
  Math Function1/1 -> Add2/2
  Add2/1 -> Gain2/1
  Gain2/1 -> Sqrt/1
  Gain/1 -> P/1
  Gain1/1 -> Q/1
  mult4/1 -> Gain3/1
  Gain3/1 -> Add/3
  Trigonometric Function/1 -> Gain4/1
  Gain4/1 -> Vph_deg/1

== system exSyncGenPVinv_sim/Photovoltaic Inverter/active power loop compensator ==
  vdc_err : Inport
  Add : Sum
  Add1 : Sum
  Constant4 : Constant  Value=Pdc_op/3
  Gain1 : Gain  Gain=Kpp
  Gain2 : Gain  Gain=Kpi
  Integrator : Integrator
  pstar : Outport
  wires:
  vdc_err/1 -> Gain2/1, Gain1/1
  Add1/1 -> Add/2
  Gain1/1 -> Add/1
  Gain2/1 -> Integrator/1
  Integrator/1 -> Add1/1
  Constant4/1 -> Add1/2
  Add/1 -> pstar/1

== system exSyncGenPVinv_sim/Photovoltaic Inverter/bridge input dc power discharging the bus capacitor ==
  idq : Inport
  vdq_inv : Inport  Port=2
  Add : Sum
  Demux : Demux  Outputs=2
  Demux1 : Demux  Outputs=2
  Gain : Gain  Gain=3/2
  mult : Product  Inputs=**
  mult1 : Product  Inputs=**
  pinv (3ph) : Outport
  wires:
  idq/1 -> Demux1/1
  vdq_inv/1 -> Demux/1
  Demux/1 -> mult/1  "vd_inv"
  Demux/2 -> mult1/1  "vq_inv"
  Demux1/1 -> mult/2  "id"
  Demux1/2 -> mult1/2  "iq"
  mult/1 -> Add/1
  mult1/1 -> Add/2
  Add/1 -> Gain/1
  Gain/1 -> pinv (3ph)/1

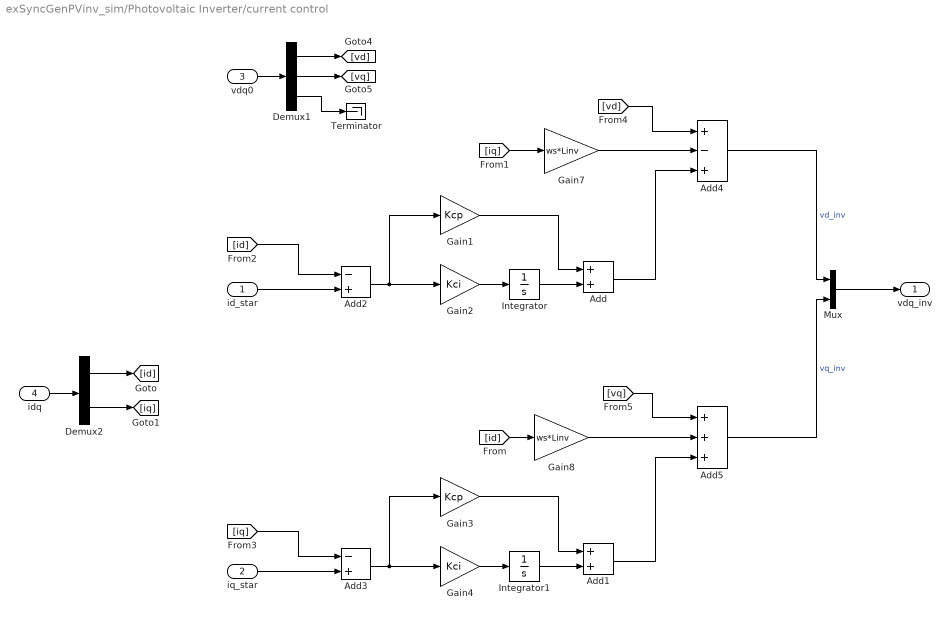
== system exSyncGenPVinv_sim/Photovoltaic Inverter/current control ==
  id_star : Inport
  iq_star : Inport  Port=2
  vdq0 : Inport  Port=3
  idq : Inport  Port=4
  Add : Sum
  Add1 : Sum
  Add2 : Sum  Inputs=-+
  Add3 : Sum  Inputs=-+
  Add4 : Sum  Inputs=+-+
  Add5 : Sum  Inputs=+++
  Demux1 : Demux  Outputs=3
  Demux2 : Demux  Outputs=2
  Gain1 : Gain  Gain=Kcp
  Gain2 : Gain  Gain=Kci
  Gain3 : Gain  Gain=Kcp
  Gain4 : Gain  Gain=Kci
  Gain7 : Gain  Gain=ws*Linv
  Gain8 : Gain  Gain=ws*Linv
  Integrator : Integrator
  Integrator1 : Integrator
  Mux : Mux  Inputs=2
  Terminator : Terminator
  vdq_inv : Outport
  wires:
  Add2/1 -> Gain2/1, Gain1/1
  Integrator/1 -> Add/2
  Add/1 -> Add4/3
  Gain1/1 -> Add/1
  Gain2/1 -> Integrator/1
  Add3/1 -> Gain4/1, Gain3/1
  Integrator1/1 -> Add1/2
  Add1/1 -> Add5/3
  Gain3/1 -> Add1/1
  Gain4/1 -> Integrator1/1
  Add4/1 -> Mux/1  "vd_inv"
  Add5/1 -> Mux/2  "vq_inv"
  id_star/1 -> Add2/2
  iq_star/1 -> Add3/2
  [vd] -> Add4/1
  [vq] -> Add5/1
  Gain7/1 -> Add4/2
  [iq] -> Gain7/1
  Gain8/1 -> Add5/2
  [id] -> Gain8/1
  Mux/1 -> vdq_inv/1
  Demux1/3 -> Terminator/1
  Demux1/2 -> [vq]
  Demux1/1 -> [vd]
  vdq0/1 -> Demux1/1
  Demux2/2 -> [iq]
  Demux2/1 -> [id]
  idq/1 -> Demux2/1
  [id] -> Add2/1
  [iq] -> Add3/1

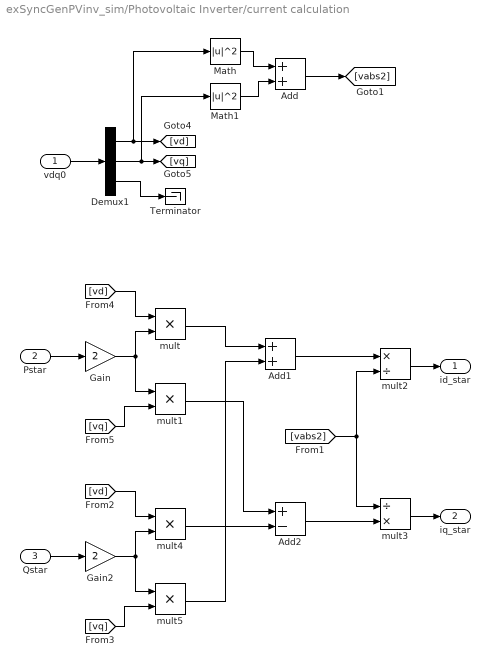
== system exSyncGenPVinv_sim/Photovoltaic Inverter/current calculation ==
  vdq0 : Inport
  Pstar : Inport  Port=2
  Qstar : Inport  Port=3
  Add : Sum
  Add1 : Sum
  Add2 : Sum  Inputs=+-
  Demux1 : Demux  Outputs=3
  Gain : Gain  Gain=2
  Gain2 : Gain  Gain=2
  Math : Math  Operator=magnitude^2  SaturateOnIntegerOverflow=on
  Math1 : Math  Operator=magnitude^2  SaturateOnIntegerOverflow=on
  Terminator : Terminator
  mult{,1,4..5} (4 alike) : Product  Inputs=**
  mult2 : Product  Inputs=*/
  mult3 : Product  Inputs=/*
  id_star : Outport
  iq_star : Outport  Port=2
  wires:
  Demux1/3 -> Terminator/1
  Demux1/2 -> Math1/1, [vq]
  Demux1/1 -> Math/1, [vd]
  vdq0/1 -> Demux1/1
  Math/1 -> Add/1
  Math1/1 -> Add/2
  Add/1 -> [vabs2]
  Pstar/1 -> Gain/1
  Gain/1 -> mult1/1, mult/2
  [vd] -> mult/1
  [vq] -> mult1/2
  Qstar/1 -> Gain2/1
  Gain2/1 -> mult5/1, mult4/2
  [vd] -> mult4/1
  [vq] -> mult5/2
  mult2/1 -> id_star/1
  [vabs2] -> mult3/1, mult2/2
  mult3/1 -> iq_star/1
  Add1/1 -> mult2/1
  mult/1 -> Add1/1
  mult5/1 -> Add1/2
  mult4/1 -> Add2/2
  mult1/1 -> Add2/1
  Add2/1 -> mult3/2

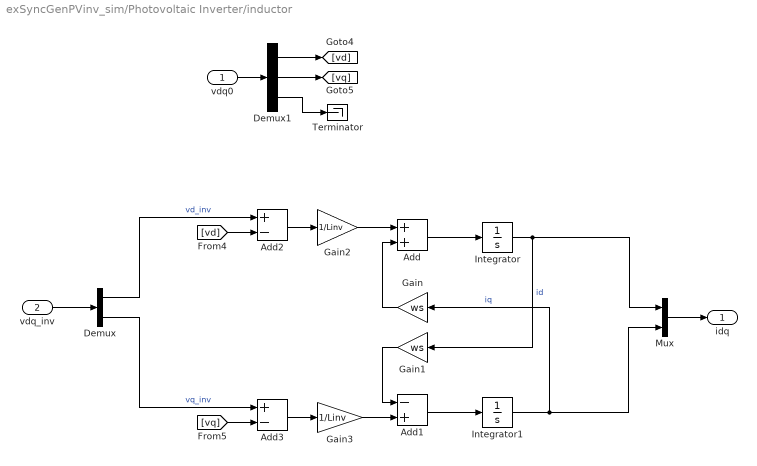
== system exSyncGenPVinv_sim/Photovoltaic Inverter/inductor ==
  vdq0 : Inport
  vdq_inv : Inport  Port=2
  Add : Sum
  Add1 : Sum  Inputs=-+
  Add2 : Sum  Inputs=+-
  Add3 : Sum  Inputs=+-
  Demux : Demux  Outputs=2
  Demux1 : Demux  Outputs=3
  Gain : Gain  Gain=ws
  Gain1 : Gain  Gain=ws
  Gain2 : Gain  Gain=1/Linv
  Gain3 : Gain  Gain=1/Linv
  Integrator : Integrator  InitialCondition=(2^0.5)*(Pdc_op/3)/Vinv_rt
  Integrator1 : Integrator
  Mux : Mux  Inputs=2
  Terminator : Terminator
  idq : Outport
  wires:
  Integrator/1 -> Gain1/1, Mux/1  "id"
  Integrator1/1 -> Mux/2, Gain/1  "iq"
  Add/1 -> Integrator/1
  Add1/1 -> Integrator1/1
  Gain/1 -> Add/2
  Gain1/1 -> Add1/1
  Gain2/1 -> Add/1
  Gain3/1 -> Add1/2
  Demux/1 -> Add2/1  "vd_inv"
  Add2/1 -> Gain2/1
  Add3/1 -> Gain3/1
  Demux/2 -> Add3/1  "vq_inv"
  [vd] -> Add2/2
  [vq] -> Add3/2
  vdq_inv/1 -> Demux/1
  vdq0/1 -> Demux1/1
  Demux1/1 -> [vd]
  Demux1/3 -> Terminator/1
  Demux1/2 -> [vq]
  Mux/1 -> idq/1
